simulink model "flags_task"  (Simulink 3.00)
libraries: inoutlib x6, mathlib x1

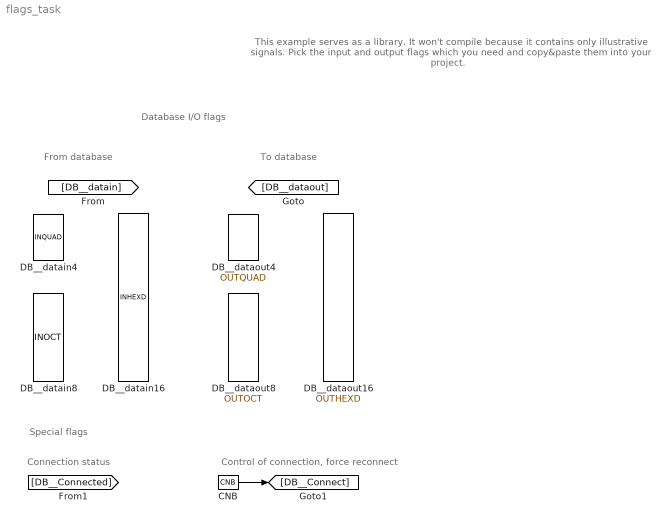
== system flags_task ==
  note: Database I/O flags
  note: From database
  note: To database
  note: Special flags
  note: Connection status
  note: Control of connection, force reconnect
  note: This example serves as a library. It won't compile because it contains only illustrative signals.
      |
      | Pick the input and output flags which you need and copy&paste them into your project.
  CNB : mathlib/CNB  YCN=on
  DB__datain16 : inoutlib/INHEXD
  DB__datain4 : inoutlib/INQUAD
  DB__datain8 : inoutlib/INOCT
  DB__dataout16 : inoutlib/OUTHEXD
  DB__dataout4 : inoutlib/OUTQUAD
  DB__dataout8 : inoutlib/OUTOCT
  wires:
  CNB/1 -> [DB__Connect]
